simulink model "emptytemplate"  (R2013a)
settings: Solver=ode4  StartTime=0.0  StopTime=inf  FixedStep=0.001  RelTol=1e-3
libraries: opal_lib x3, rtlab x2, simulink x1
Description:
  | Model of a simple control system for use iin training.
settings Model: Creator=Paul Baracos  LastModifiedBy=adam_
settings DataIOCC: SignalLoggingSaveFormat=ModelDataLogs  SaveOutput=off  SaveTime=off  SignalLoggingName=sigsOut
settings OptimizationCC: BlockReduction=off  BooleanDataType=off  OptimizeBlockIOStorage=off  BufferReuse=off  ExpressionFolding=off  LocalBlockOutputs=off  InitFltsAndDblsToZero=on
settings DebuggingCC: SaveWithParameterizedLinksMsg=none  SignalResolutionControl=TryResolveAllWithWarning  SolverPrmCheckMsg=none  MultiTaskDSMMsg=warning  MultiTaskCondExecSysMsg=none  FcnCallInpInsideContextMsg=EnableAllAsWarning  FrameProcessingCompatibilityMsg=error  StateNameClashWarn=none
settings HardwareCC: TargetUnknown=on
settings GRTTargetCC: TargetFcnLib=ansi_tfl_tmw.mat  CodeReplacementLibrary=C89/C90 (ANSI)  CombineOutputUpdateFcns=off  GRTInterface=on

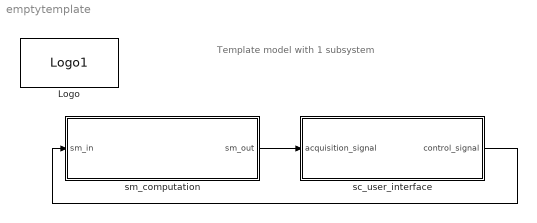
== system emptytemplate ==
  note: Template model with 1 subsystem
  Logo : opal_lib/Logo1  vide=[]
  sc_user_interface : Subsystem
  sm_computation : Subsystem
  wires:
  sc_user_interface/1(control_signal) -> sm_computation/1(sm_in)
  sm_computation/1(sm_out) -> sc_user_interface/1(acquisition_signal)

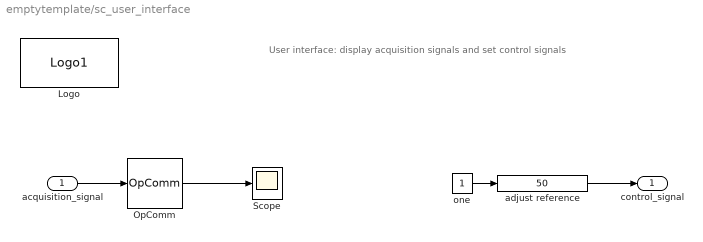
== system emptytemplate/sc_user_interface ==
  note: User interface: display acquisition signals and set control signals
  acquisition_signal : Inport
  Logo : opal_lib/Logo1  vide=[]
  OpComm : rtlab/OpComm  nbport=1  groupe_acq=1  subsys_rate=0  st=0  Synchronization=on  Interpolation=on  Threshold=1.0  Missed_Data=off  Sim_Time=off  Samples=off  dynSigOut=off  from_console=0  warning_done=off  writeOpCommFile=off  Offset=off
  Scope : Scope
      settings: Tag=op_tm_save_it  TimeRange=10  LimitDataPoints=on  MaxDataPoints=5000  SaveToWorkspace=off  SaveName=referenceAndPlant  YMin=0  YMax=100  SampleTime=-1
  adjust reference : simulink/Math Operations/Slider Gain  gain=50  low=0  high=100
  one : Constant
  control_signal : Outport
  wires:
  acquisition_signal/1 -> OpComm/1
  OpComm/1 -> Scope/1
  adjust reference/1 -> control_signal/1
  one/1 -> adjust reference/1

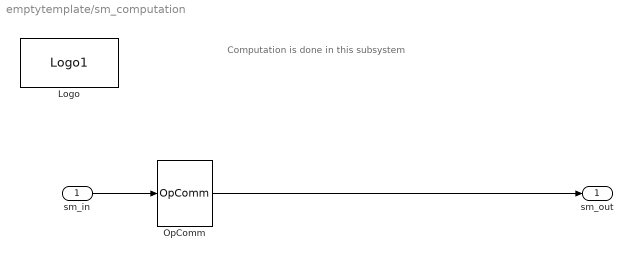
== system emptytemplate/sm_computation ==
  note: Computation is done in this subsystem
  sm_in : Inport
  Logo : opal_lib/Logo1  vide=[]
  OpComm : rtlab/OpComm  nbport=1  groupe_acq=1  subsys_rate=0  st=0  Synchronization=on  Interpolation=on  Threshold=1.0  Missed_Data=off  Sim_Time=off  Samples=off  dynSigOut=off  from_console=1  warning_done=off  writeOpCommFile=off  Offset=off
  sm_out : Outport
  wires:
  sm_in/1 -> OpComm/1
  OpComm/1 -> sm_out/1
